simulink model "OneOneTwo"  (R2022b)
settings: Solver=VariableStepAuto  StartTime=0.0  StopTime=10.0  RelTol=1e-3
settings Model: Creator=yeyi5  LastModifiedBy=yeyi5
settings DataIOCC: ReturnWorkspaceOutputs=off

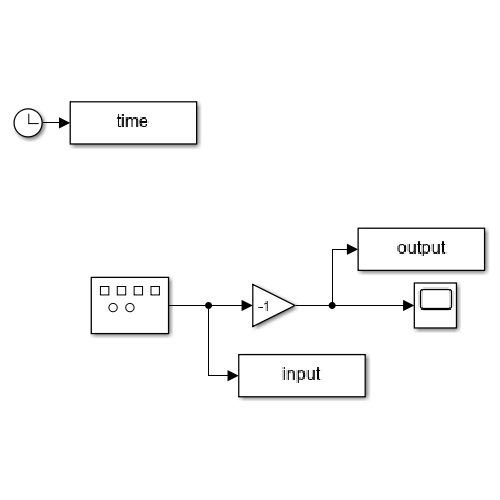
[thumbnail: Simulink's stored preview of the top-level diagram]
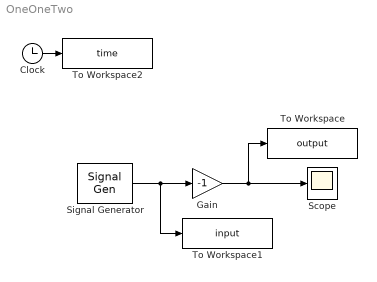
== system OneOneTwo ==
  Clock : Clock
  Gain : Gain  Gain=-1
  Scope : Scope
  Signal Generator : SignalGenerator  WaveForm=square  Amplitude=2  Frequency=0.5
  To Workspace : ToWorkspace  VariableName=output  SampleTime=-1
  To Workspace1 : ToWorkspace  VariableName=input  SampleTime=-1
  To Workspace2 : ToWorkspace  VariableName=time  SampleTime=-1
  wires:
  Signal Generator/1 -> To Workspace1/1, Gain/1
  Gain/1 -> To Workspace/1, Scope/1
  Clock/1 -> To Workspace2/1
